simulink library "Lib_HStab"  (R2018b)
settings: Solver=VariableStepAuto  StartTime=0.0  StopTime=10.0  RelTol=1e-3
values from neighbouring files (symbols this model uses):
  AutoTrim_On = 1    [SimulationHStabConfig.m]
  dt = DLLSim.dt    [SimulationTimeStep.m]    (also in SimulationTrim.m = 0.02)
  HStab = 0    [SimulationAircraftConfig.m]
  HStab_Offset = 0    [SimulationHStabConfig.m]
undefined symbols (not defined in the file or in its folder): DiscIntNeverNeededParam, HStabSystem, Trim_REFSI_FD_IN_nmodeStabCmd
libraries: simulink x14, $bdroot x2
settings Model: Creator=JCdFFigueira  LastModifiedBy=JFigueira-Admin
settings DataIOCC: ReturnWorkspaceOutputs=on
settings DebuggingCC: UnconnectedInputMsg=none  UnconnectedOutputMsg=none  UnconnectedLineMsg=none
settings ModelReferenceCC: EnableRefExpFcnMdlSchedulingChecks=off
settings RTWCC: Description=Generic Real-Time Target

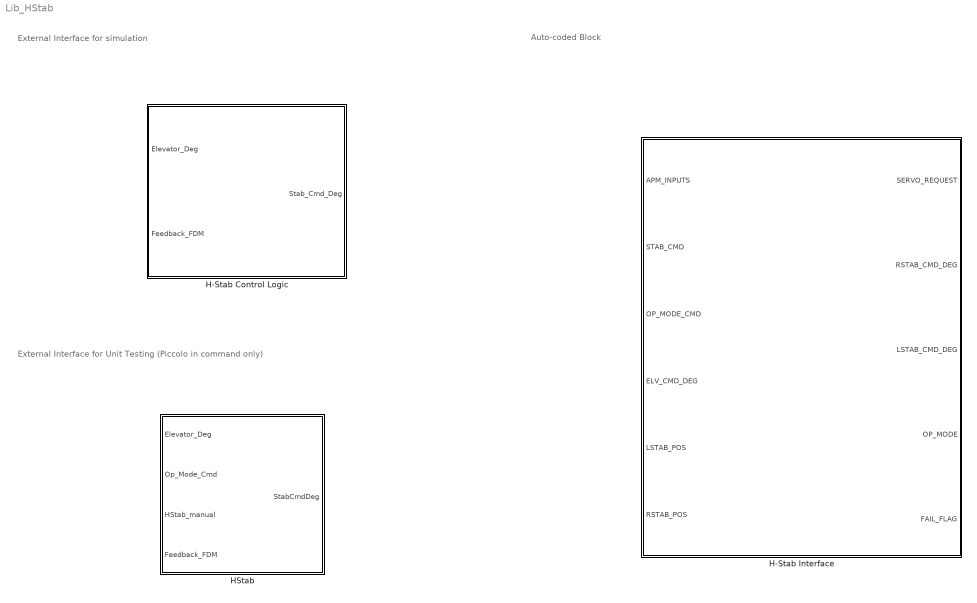
== system Lib_HStab ==
  note: External Interface for Unit Testing (Piccolo in command only)
  note: External Interface for simulation
  note: Auto-coded Block
  H-Stab Control Logic : Subsystem  Variant=on  VariantControl=Variant1
  H-Stab Interface : Subsystem  TreatAsAtomicUnit=on  SystemSampleTime=0.02
  HStab : Subsystem

== system Lib_HStab/H-Stab Control Logic ==
  "Elevator_Deg " : Inport
  Feedback_FDM : Inport  Port=2
  H-Stab Control Logic : Subsystem  VariantControl=FTV == 4 && FDMRelease >= 40
  H-Stab Placeholder : Subsystem  VariantControl=FTV == 3 || FDMRelease < 40
  " Stab_Cmd_Deg" : Outport

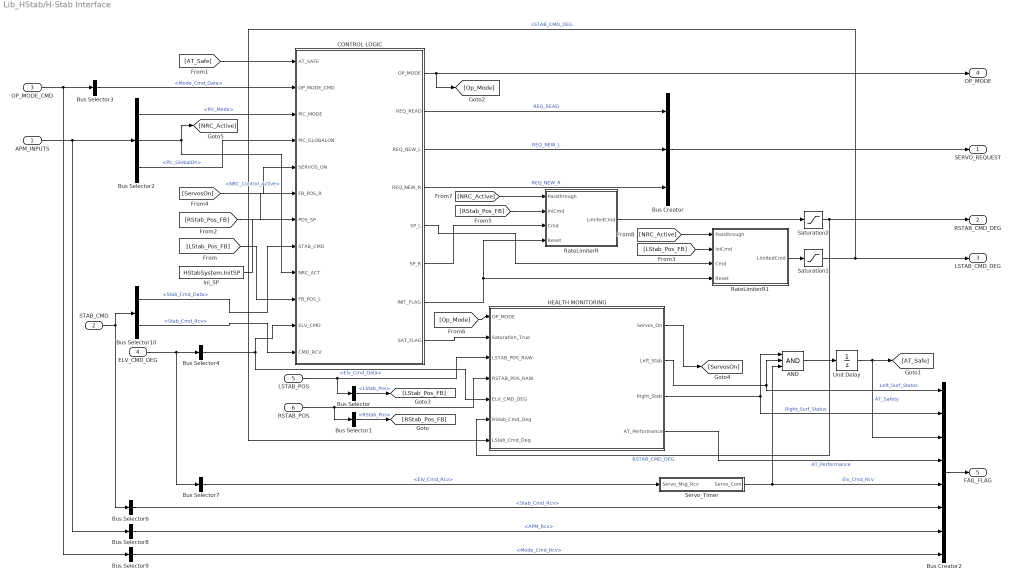
== system Lib_HStab/H-Stab Interface ==
  APM_INPUTS : Inport  OutDataTypeStr=Bus: APM_Bus
  STAB_CMD : Inport  Port=2  OutDataTypeStr=Bus: HStab_Cmd  LockScale=on
  OP_MODE_CMD : Inport  Port=3  OutDataTypeStr=Bus: Mode_Cmd
  ELV_CMD_DEG : Inport  Port=4  OutDataTypeStr=Bus: ELV_Cmd  LockScale=on
  LSTAB_POS : Inport  Port=5  OutDataTypeStr=Bus: LServo_FB  LockScale=on
  RSTAB_POS : Inport  Port=6  OutDataTypeStr=Bus: RServo_FB  LockScale=on
  AND : Logic  Inputs=3  IconShape=distinctive  AllPortsSameDT=off  OutDataTypeStr=boolean
  Bus Creator : BusCreator  Inputs=3
  Bus Creator2 : BusCreator  Inputs=8
  Bus Selector : BusSelector  OutputSignals=LStab_Pos
  Bus Selector1 : BusSelector  OutputSignals=RStab_Pos
  Bus Selector10 : BusSelector  OutputSignals=Stab_Cmd_Data,Stab_Cmd_Rcv
  Bus Selector2 : BusSelector  OutputSignals=Pic_Mode,NRC_Control_Active,Pic_GlobalOn
  Bus Selector3 : BusSelector  OutputSignals=Mode_Cmd_Data
  Bus Selector4 : BusSelector  OutputSignals=Elv_Cmd_Data
  Bus Selector6 : BusSelector  OutputSignals=Stab_Cmd_Rcv
  Bus Selector7 : BusSelector  OutputSignals=Elv_Cmd_Rcv
  Bus Selector8 : BusSelector  OutputSignals=APM_Rcv
  Bus Selector9 : BusSelector  OutputSignals=Mode_Cmd_Rcv
  CONTROL LOGIC : Stateflow chart  TreatAsAtomicUnit=on  SystemSampleTime=0.02
  HEALTH MONITORING : Subsystem
  Ini_SP : Constant  Value=HStabSystem.InitSP  OutDataTypeStr=single
  RateLimiterR : Subsystem
  RateLimiterR1 : Subsystem
  Saturation1 : Saturate  UpperLimit=HStabSystem.LimitUpper  LowerLimit=HStabSystem.LimitLower  OutDataTypeStr=single
  Saturation2 : Saturate  UpperLimit=HStabSystem.LimitUpper  LowerLimit=HStabSystem.LimitLower  OutDataTypeStr=single
  Servo_Timer : Subsystem
  Unit Delay : UnitDelay  InitialCondition=1  SampleTime=0.02
  SERVO_REQUEST : Outport  OutDataTypeStr=Bus: Servo_Request  SampleTime=0.02  VectorParamsAs1DForOutWhenUnconnected=on
  RSTAB_CMD_DEG : Outport  Port=2  OutDataTypeStr=single  VectorParamsAs1DForOutWhenUnconnected=on
  LSTAB_CMD_DEG : Outport  Port=3  OutDataTypeStr=single  VectorParamsAs1DForOutWhenUnconnected=on
  OP_MODE : Outport  Port=4  OutDataTypeStr=uint8  VectorParamsAs1DForOutWhenUnconnected=on
  FAIL_FLAG : Outport  Port=5  OutDataTypeStr=Bus: Fail_Flag_Bus  VectorParamsAs1DForOutWhenUnconnected=on
  wires:
  Saturation1/1 -> LSTAB_CMD_DEG/1, HEALTH MONITORING/7(LStab_Cmd_Deg)  "LSTAB_CMD_DEG"
  Saturation2/1 -> RSTAB_CMD_DEG/1, HEALTH MONITORING/6(RStab_Cmd_Deg)  "RSTAB_CMD_DEG"
  RateLimiterR/1(LimitedCmd) -> Saturation2/1
  [RStab_Pos_FB] -> RateLimiterR/2(IniCmd)
  [LStab_Pos_FB] -> RateLimiterR1/2(IniCmd)
  [RStab_Pos_FB] -> CONTROL LOGIC/6(FB_POS_R)
  [LStab_Pos_FB] -> CONTROL LOGIC/10(FB_POS_L)
  Bus Selector1/1 -> [RStab_Pos_FB]  "<RStab_Pos>"
  Bus Selector/1 -> [LStab_Pos_FB]  "<LStab_Pos>"
  CONTROL LOGIC/7(INIT_FLAG) -> RateLimiterR/4(Reset), RateLimiterR1/4(Reset)
  RateLimiterR1/1(LimitedCmd) -> Saturation1/1
  CONTROL LOGIC/5(SP_L) -> RateLimiterR1/3(Cmd)
  CONTROL LOGIC/6(SP_R) -> RateLimiterR/3(Cmd)
  [ServosOn] -> CONTROL LOGIC/5(SERVOS_ON)
  HEALTH MONITORING/1(Servos_On) -> [ServosOn]
  STAB_CMD/1 -> Bus Selector6/1, Bus Selector10/1
  Ini_SP/1 -> CONTROL LOGIC/7(POS_SP)
  Bus Creator/1 -> SERVO_REQUEST/1
  ELV_CMD_DEG/1 -> Bus Selector7/1, Bus Selector4/1
  CONTROL LOGIC/1(OP_MODE) -> OP_MODE/1, [Op_Mode]
  RSTAB_POS/1 -> HEALTH MONITORING/4(RSTAB_POS_RAW), Bus Selector1/1
  LSTAB_POS/1 -> HEALTH MONITORING/3(LSTAB_POS_RAW), Bus Selector/1
  OP_MODE_CMD/1 -> Bus Selector9/1, Bus Selector3/1
  APM_INPUTS/1 -> Bus Selector8/1, Bus Selector2/1
  HEALTH MONITORING/3(Right_Stab) -> Bus Creator2/2, AND/1  "Right_Surf_Status"
  HEALTH MONITORING/2(Left_Stab) -> Bus Creator2/1, AND/2  "Left_Surf_Status"
  Bus Creator2/1 -> FAIL_FLAG/1
  CONTROL LOGIC/8(SAT_FLAG) -> HEALTH MONITORING/2(Saturation_True)
  HEALTH MONITORING/4(AT_Performance) -> Bus Creator2/4  "AT_Performance"
  Bus Selector2/1 -> CONTROL LOGIC/3(PIC_MODE)  "<Pic_Mode>"
  Bus Selector2/2 -> CONTROL LOGIC/9(NRC_ACT), [NRC_Active]  "<NRC_Control_Active>"
  Bus Selector2/3 -> CONTROL LOGIC/4(PIC_GLOBALON)  "<Pic_GlobalOn>"
  Bus Selector3/1 -> CONTROL LOGIC/2(OP_MODE_CMD)  "<Mode_Cmd_Data>"
  Bus Selector4/1 -> HEALTH MONITORING/5(ELV_CMD_DEG), CONTROL LOGIC/11(ELV_CMD)  "<Elv_Cmd_Data>"
  Bus Selector6/1 -> Bus Creator2/6  "<Stab_Cmd_Rcv>"
  Bus Selector8/1 -> Bus Creator2/7  "<APM_Rcv>"
  Bus Selector9/1 -> Bus Creator2/8  "<Mode_Cmd_Rcv>"
  CONTROL LOGIC/2(REQ_READ) -> Bus Creator/1  "REQ_READ"
  CONTROL LOGIC/3(REQ_NEW_L) -> Bus Creator/2  "REQ_NEW_L"
  CONTROL LOGIC/4(REQ_NEW_R) -> Bus Creator/3  "REQ_NEW_R"
  AND/1 -> Unit Delay/1
  [AT_Safe] -> CONTROL LOGIC/1(AT_SAFE)
  Unit Delay/1 -> Bus Creator2/3, [AT_Safe]  "AT_Safety"
  Bus Selector10/1 -> CONTROL LOGIC/8(STAB_CMD)  "<Stab_Cmd_Data>"
  [Op_Mode] -> HEALTH MONITORING/1(OP_MODE)
  [NRC_Active] -> RateLimiterR/1(Passthrough)
  [NRC_Active] -> RateLimiterR1/1(Passthrough)
  Bus Selector10/2 -> CONTROL LOGIC/12(CMD_RCV)  "<Stab_Cmd_Rcv>"
  Servo_Timer/1(Servo_Com) -> AND/3, Bus Creator2/5  "Elv_Cmd_Rcv"
  Bus Selector7/1 -> Servo_Timer/1(Servo_Msg_Rcv)  "<Elv_Cmd_Rcv>"

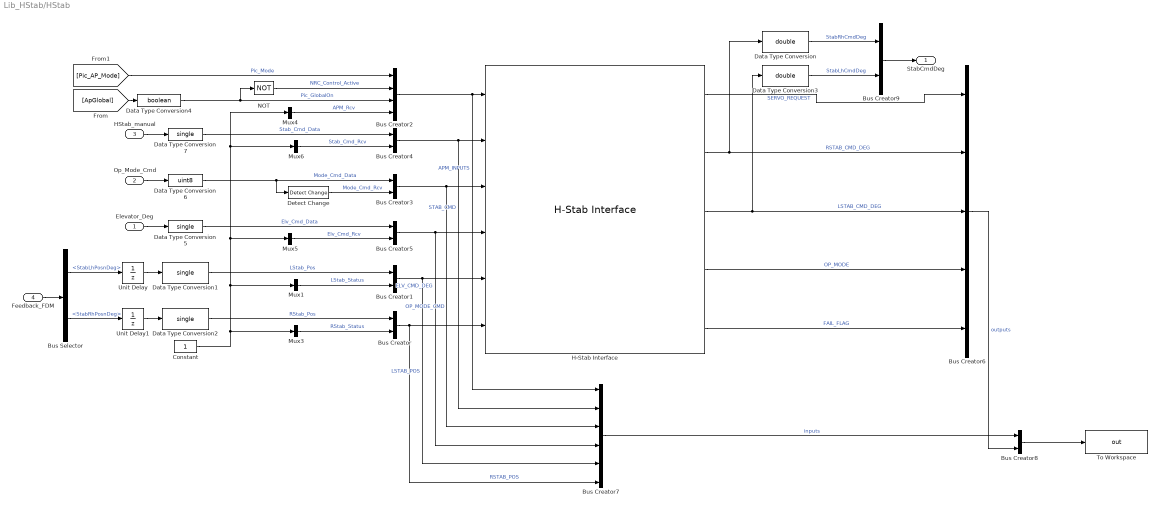
== system Lib_HStab/HStab ==
  Elevator_Deg : Inport  OutDataTypeStr=single  LockScale=on
  Op_Mode_Cmd : Inport  Port=2  OutDataTypeStr=uint8  LockScale=on
  HStab_manual : Inport  Port=3  OutDataTypeStr=single  LockScale=on
  Feedback_FDM : Inport  Port=4
  Bus Creator{,1,3..5,8..9} (7 alike) : BusCreator  Inputs=2
  Bus Creator2 : BusCreator  Inputs=4
  Bus Creator6 : BusCreator  Inputs=5
  Bus Creator7 : BusCreator  Inputs=6
  Bus Selector : BusSelector  OutputSignals=StabLhPosnDeg,StabRhPosnDeg
  Constant : Constant  OutDataTypeStr=boolean
  Data Type Conversion : DataTypeConversion  OutDataTypeStr=double
  Data Type Conversion{1..2,5,7} (4 alike) : DataTypeConversion  OutDataTypeStr=single
  Data Type Conversion3 : DataTypeConversion  OutDataTypeStr=double
  Data Type Conversion4 : DataTypeConversion  OutDataTypeStr=boolean
  Data Type Conversion6 : DataTypeConversion  OutDataTypeStr=uint8
  Detect Change : simulink/Logic and Bit Operations/Detect Change  vinit=2  OutDataTypeStr=boolean
  H-Stab Interface : $bdroot/H-Stab Interface  SystemSampleTime=0.02
  Mux{1,3..6} (5 alike) : Mux  Inputs=1
  NOT : Logic  Operator=NOT  IconShape=distinctive  AllPortsSameDT=off  OutDataTypeStr=boolean
  To Workspace : ToWorkspace  VariableName=out  SaveFormat=Timeseries  SampleTime=dt
  Unit Delay : UnitDelay  InitialCondition=HStab  SampleTime=dt
  Unit Delay1 : UnitDelay  InitialCondition=HStab  SampleTime=dt
  StabCmdDeg : Outport  OutDataTypeStr=double  VectorParamsAs1DForOutWhenUnconnected=on
  wires:
  Data Type Conversion4/1 -> NOT/1, Bus Creator2/3  "Pic_GlobalOn"
  [Pic_AP_Mode] -> Bus Creator2/1  "Pic_Mode"
  Data Type Conversion5/1 -> Bus Creator5/1  "Elv_Cmd_Data"
  Data Type Conversion7/1 -> Bus Creator4/1  "Stab_Cmd_Data"
  Data Type Conversion1/1 -> Bus Creator1/1  "LStab_Pos"
  Mux1/1 -> Bus Creator1/2  "LStab_Status"
  Data Type Conversion2/1 -> Bus Creator/1  "RStab_Pos"
  Mux3/1 -> Bus Creator/2  "RStab_Status"
  Constant/1 -> Mux3/1, Mux1/1, Mux5/1, Mux6/1, Mux4/1
  NOT/1 -> Bus Creator2/2  "NRC_Control_Active"
  Data Type Conversion6/1 -> Detect Change/1, Bus Creator3/1  "Mode_Cmd_Data"
  Mux4/1 -> Bus Creator2/4  "APM_Rcv"
  Mux5/1 -> Bus Creator5/2  "Elv_Cmd_Rcv"
  Mux6/1 -> Bus Creator4/2  "Stab_Cmd_Rcv"
  Detect Change/1 -> Bus Creator3/2  "Mode_Cmd_Rcv"
  Unit Delay/1 -> Data Type Conversion1/1
  H-Stab Interface/2 -> Bus Creator6/2, Data Type Conversion/1  "RSTAB_CMD_DEG"
  H-Stab Interface/1 -> Bus Creator6/1  "SERVO_REQUEST"
  H-Stab Interface/4 -> Bus Creator6/4  "OP_MODE"
  H-Stab Interface/3 -> Bus Creator6/3, Data Type Conversion3/1  "LSTAB_CMD_DEG"
  Bus Creator6/1 -> Bus Creator8/2  "outputs"
  H-Stab Interface/5 -> Bus Creator6/5  "FAIL_FLAG"
  Bus Creator1/1 -> H-Stab Interface/5, Bus Creator7/5  "LSTAB_POS"
  Bus Creator3/1 -> H-Stab Interface/3, Bus Creator7/3  "OP_MODE_CMD"
  Bus Creator5/1 -> H-Stab Interface/4, Bus Creator7/4  "ELV_CMD_DEG"
  Bus Creator4/1 -> H-Stab Interface/2, Bus Creator7/2  "STAB_CMD"
  Bus Creator7/1 -> Bus Creator8/1  "inputs"
  Bus Creator/1 -> H-Stab Interface/6, Bus Creator7/6  "RSTAB_POS"
  Bus Creator2/1 -> H-Stab Interface/1, Bus Creator7/1  "APM_INPUTS"
  Unit Delay1/1 -> Data Type Conversion2/1
  Data Type Conversion/1 -> Bus Creator9/1  "StabRhCmdDeg"
  Data Type Conversion3/1 -> Bus Creator9/2  "StabLhCmdDeg"
  Bus Creator8/1 -> To Workspace/1
  Bus Creator9/1 -> StabCmdDeg/1
  [ApGlobal] -> Data Type Conversion4/1
  Elevator_Deg/1 -> Data Type Conversion5/1
  Op_Mode_Cmd/1 -> Data Type Conversion6/1
  HStab_manual/1 -> Data Type Conversion7/1
  Feedback_FDM/1 -> Bus Selector/1
  Bus Selector/1 -> Unit Delay/1  "<StabLhPosnDeg>"
  Bus Selector/2 -> Unit Delay1/1  "<StabRhPosnDeg>"

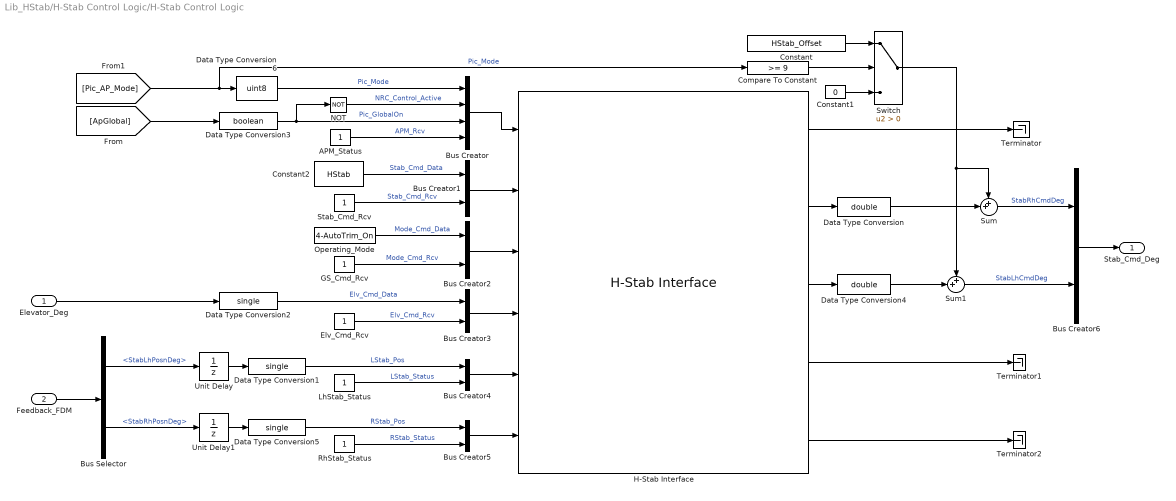
== system Lib_HStab/H-Stab Control Logic/H-Stab Control Logic ==
  Elevator_Deg : Inport
  Feedback_FDM : Inport  Port=2
  APM_Status : Constant  OutDataTypeStr=boolean
  Bus Creator : BusCreator  Inputs=4
  Bus Creator{1..6} (6 alike) : BusCreator  Inputs=2
  Bus Selector : BusSelector  OutputSignals=StabLhPosnDeg,StabRhPosnDeg
  Compare To Constant : simulink/Logic and Bit Operations/Compare To Constant  relop=>=  const=9  OutDataTypeStr=boolean
  Constant : Constant  Value=HStab_Offset  OutDataTypeStr=double
  Constant1 : Constant  Value=0  OutDataTypeStr=double
  Constant2 : Constant  Value=HStab  OutDataTypeStr=single
  Data Type Conversion : DataTypeConversion  OutDataTypeStr=double  LockScale=on
  Data Type Conversion1 : DataTypeConversion  OutDataTypeStr=single
  Data Type Conversion2 : DataTypeConversion  OutDataTypeStr=single
  Data Type Conversion3 : DataTypeConversion  OutDataTypeStr=boolean
  Data Type Conversion4 : DataTypeConversion  OutDataTypeStr=double  LockScale=on
  Data Type Conversion5 : DataTypeConversion  OutDataTypeStr=single
  Data Type Conversion6 : DataTypeConversion  OutDataTypeStr=uint8
  Elv_Cmd_Rcv : Constant  OutDataTypeStr=boolean
  GS_Cmd_Rcv : Constant  OutDataTypeStr=boolean
  H-Stab Interface : $bdroot/H-Stab Interface  SystemSampleTime=0.02
  LhStab_Status : Constant  OutDataTypeStr=boolean
  NOT : Logic  Operator=NOT  IconShape=distinctive  AllPortsSameDT=off  OutDataTypeStr=boolean
  Operating_Mode : Constant  Value=4-AutoTrim_On  OutDataTypeStr=uint8
  RhStab_Status : Constant  OutDataTypeStr=boolean
  Stab_Cmd_Rcv : Constant  OutDataTypeStr=boolean
  Sum : Sum  Inputs=++|
  Sum1 : Sum  Inputs=++|
  Switch : Switch  Criteria=u2 > Threshold
  Terminator : Terminator
  Terminator1 : Terminator
  Terminator2 : Terminator
  Unit Delay : UnitDelay  InitialCondition=HStab  SampleTime=-1
  Unit Delay1 : UnitDelay  InitialCondition=HStab  SampleTime=-1
  Stab_Cmd_Deg : Outport
  wires:
  [Pic_AP_Mode] -> Compare To Constant/1, Data Type Conversion6/1  "Pic_Mode"
  Switch/1 -> Sum1/1, Sum/1
  Compare To Constant/1 -> Switch/2
  Constant/1 -> Switch/1
  Constant1/1 -> Switch/3
  Data Type Conversion6/1 -> Bus Creator/1  "Pic_Mode"
  [ApGlobal] -> Data Type Conversion3/1
  Unit Delay1/1 -> Data Type Conversion5/1
  Bus Selector/2 -> Unit Delay1/1  "<StabRhPosnDeg>"
  Bus Selector/1 -> Unit Delay/1  "<StabLhPosnDeg>"
  H-Stab Interface/4 -> Terminator1/1
  Bus Creator/1 -> H-Stab Interface/1
  Bus Creator4/1 -> H-Stab Interface/5
  APM_Status/1 -> Bus Creator/4  "APM_Rcv"
  RhStab_Status/1 -> Bus Creator5/2  "RStab_Status"
  H-Stab Interface/2 -> Data Type Conversion/1
  Bus Creator1/1 -> H-Stab Interface/2
  Data Type Conversion3/1 -> Bus Creator/3, NOT/1  "Pic_GlobalOn"
  H-Stab Interface/1 -> Terminator/1
  NOT/1 -> Bus Creator/2  "NRC_Control_Active"
  Bus Creator2/1 -> H-Stab Interface/3
  Elv_Cmd_Rcv/1 -> Bus Creator3/2  "Elv_Cmd_Rcv"
  H-Stab Interface/5 -> Terminator2/1
  Bus Creator5/1 -> H-Stab Interface/6
  Data Type Conversion5/1 -> Bus Creator5/1  "RStab_Pos"
  Stab_Cmd_Rcv/1 -> Bus Creator1/2  "Stab_Cmd_Rcv"
  Data Type Conversion1/1 -> Bus Creator4/1  "LStab_Pos"
  Data Type Conversion2/1 -> Bus Creator3/1  "Elv_Cmd_Data"
  Operating_Mode/1 -> Bus Creator2/1  "Mode_Cmd_Data"
  Unit Delay/1 -> Data Type Conversion1/1
  Feedback_FDM/1 -> Bus Selector/1
  GS_Cmd_Rcv/1 -> Bus Creator2/2  "Mode_Cmd_Rcv"
  Elevator_Deg/1 -> Data Type Conversion2/1
  Constant2/1 -> Bus Creator1/1  "Stab_Cmd_Data"
  LhStab_Status/1 -> Bus Creator4/2  "LStab_Status"
  Bus Creator3/1 -> H-Stab Interface/4
  H-Stab Interface/3 -> Data Type Conversion4/1
  Sum/1 -> Bus Creator6/1  "StabRhCmdDeg"
  Sum1/1 -> Bus Creator6/2  "StabLhCmdDeg"
  Bus Creator6/1 -> Stab_Cmd_Deg/1
  Data Type Conversion4/1 -> Sum1/2
  Data Type Conversion/1 -> Sum/2

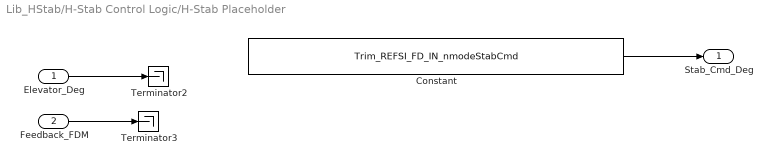
== system Lib_HStab/H-Stab Control Logic/H-Stab Placeholder ==
  Elevator_Deg : Inport
  Feedback_FDM : Inport  Port=2
  Constant : Constant  Value=Trim_REFSI_FD_IN_nmodeStabCmd
  Terminator2 : Terminator
  Terminator3 : Terminator
  Stab_Cmd_Deg : Outport
  wires:
  Constant/1 -> Stab_Cmd_Deg/1
  Elevator_Deg/1 -> Terminator2/1
  Feedback_FDM/1 -> Terminator3/1

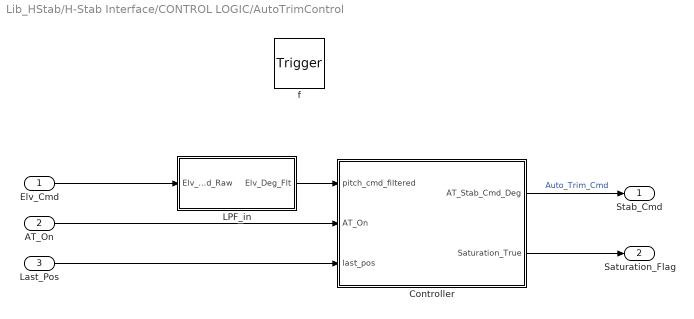
== system Lib_HStab/H-Stab Interface/CONTROL LOGIC/AutoTrimControl ==
  Elv_Cmd : Inport  OutDataTypeStr=single  PortDimensions=1
  AT_On : Inport  Port=2  OutDataTypeStr=boolean  PortDimensions=1
  Last_Pos : Inport  Port=3  OutDataTypeStr=single  PortDimensions=1
  f : TriggerPort  TriggerType=function-call  VariantControl=(inherit)
      settings: CopyFcn=Stateflow.SLINSF.SimulinkMan.removeBlockPreDeleteFcn  PreDeleteFcn=Stateflow.SLINSF.SimulinkMan.unsafePredeleteFcn
  "Controller " : Subsystem
  LPF_in : Subsystem
  Stab_Cmd : Outport  OutDataTypeStr=single  PortDimensions=1  VectorParamsAs1DForOutWhenUnconnected=on
  Saturation_Flag : Outport  Port=2  OutDataTypeStr=boolean  PortDimensions=1  VectorParamsAs1DForOutWhenUnconnected=on
  wires:
  "Controller "/2(Saturation_True) -> Saturation_Flag/1
  "Controller "/1(AT_Stab_Cmd_Deg) -> Stab_Cmd/1  "Auto_Trim_Cmd"
  Last_Pos/1 -> "Controller "/3(last_pos)
  LPF_in/1(Elv_Deg_Flt) -> "Controller "/1(pitch_cmd_filtered)
  AT_On/1 -> "Controller "/2(AT_On)
  Elv_Cmd/1 -> LPF_in/1(Elv_Cmd_Raw)

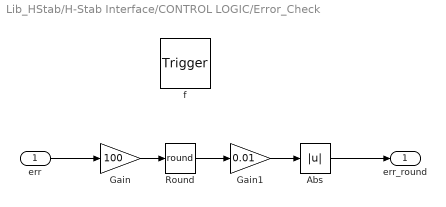
== system Lib_HStab/H-Stab Interface/CONTROL LOGIC/Error_Check ==
  err : Inport  OutDataTypeStr=single  PortDimensions=1
  f : TriggerPort  TriggerType=function-call  VariantControl=(inherit)
      settings: CopyFcn=Stateflow.SLINSF.SimulinkMan.removeBlockPreDeleteFcn  PreDeleteFcn=Stateflow.SLINSF.SimulinkMan.unsafePredeleteFcn
  Abs : Abs  OutDataTypeStr=single
  Gain : Gain  Gain=100
  Gain1 : Gain  Gain=0.01
  Round : Rounding  Operator=round
  err_round : Outport  OutDataTypeStr=single  PortDimensions=1  VectorParamsAs1DForOutWhenUnconnected=on
  wires:
  Round/1 -> Gain1/1
  Gain/1 -> Round/1
  Gain1/1 -> Abs/1
  err/1 -> Gain/1
  Abs/1 -> err_round/1

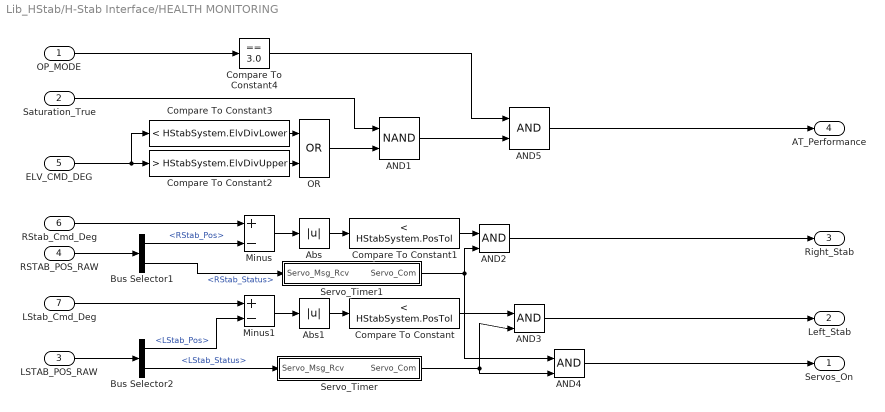
== system Lib_HStab/H-Stab Interface/HEALTH MONITORING ==
  OP_MODE : Inport  PortDimensions=1
  Saturation_True : Inport  Port=2  OutDataTypeStr=boolean  PortDimensions=1
  LSTAB_POS_RAW : Inport  Port=3  OutDataTypeStr=Bus: LServo_FB
  RSTAB_POS_RAW : Inport  Port=4  OutDataTypeStr=Bus: RServo_FB
  ELV_CMD_DEG : Inport  Port=5  OutDataTypeStr=single  PortDimensions=1
  RStab_Cmd_Deg : Inport  Port=6  OutDataTypeStr=single  PortDimensions=1
  LStab_Cmd_Deg : Inport  Port=7  OutDataTypeStr=single  PortDimensions=1
  AND1 : Logic  Operator=NAND  IconShape=distinctive  AllPortsSameDT=off  OutDataTypeStr=boolean
  AND{2..5} (4 alike) : Logic  IconShape=distinctive  AllPortsSameDT=off  OutDataTypeStr=boolean
  Abs : Abs  OutDataTypeStr=single
  Abs1 : Abs  OutDataTypeStr=single
  Bus Selector1 : BusSelector  OutputSignals=RStab_Pos,RStab_Status
  Bus Selector2 : BusSelector  OutputSignals=LStab_Pos,LStab_Status
  Compare To Constant : simulink/Logic and Bit Operations/Compare To Constant  relop=<  const=HStabSystem.PosTol  OutDataTypeStr=boolean
  Compare To Constant1 : simulink/Logic and Bit Operations/Compare To Constant  relop=<  const=HStabSystem.PosTol  OutDataTypeStr=boolean
  Compare To Constant2 : simulink/Logic and Bit Operations/Compare To Constant  relop=>  const=HStabSystem.ElvDivUpper  OutDataTypeStr=boolean
  Compare To Constant3 : simulink/Logic and Bit Operations/Compare To Constant  relop=<  const=HStabSystem.ElvDivLower  OutDataTypeStr=boolean
  Compare To Constant4 : simulink/Logic and Bit Operations/Compare To Constant  relop===  const=3.0  OutDataTypeStr=boolean
  Minus : Sum  Inputs=+-
  Minus1 : Sum  Inputs=+-
  OR : Logic  Operator=OR  IconShape=distinctive  AllPortsSameDT=off  OutDataTypeStr=boolean
  Servo_Timer : Subsystem
  Servo_Timer1 : Subsystem
  Servos_On : Outport  OutDataTypeStr=boolean  PortDimensions=1  VectorParamsAs1DForOutWhenUnconnected=on
  Left_Stab : Outport  Port=2  OutDataTypeStr=boolean  PortDimensions=1  VectorParamsAs1DForOutWhenUnconnected=on
  Right_Stab : Outport  Port=3  OutDataTypeStr=boolean  PortDimensions=1  VectorParamsAs1DForOutWhenUnconnected=on
  AT_Performance : Outport  Port=4  OutDataTypeStr=boolean  PortDimensions=1  VectorParamsAs1DForOutWhenUnconnected=on
  wires:
  Bus Selector1/2 -> Servo_Timer1/1(Servo_Msg_Rcv)  "<RStab_Status>"
  Bus Selector2/2 -> Servo_Timer/1(Servo_Msg_Rcv)  "<LStab_Status>"
  Servo_Timer/1(Servo_Com) -> AND4/2, AND3/2
  AND4/1 -> Servos_On/1
  LStab_Cmd_Deg/1 -> Minus1/1
  RStab_Cmd_Deg/1 -> Minus/1
  Servo_Timer1/1(Servo_Com) -> AND4/1, AND2/2
  LSTAB_POS_RAW/1 -> Bus Selector2/1
  RSTAB_POS_RAW/1 -> Bus Selector1/1
  Compare To Constant/1 -> AND3/1
  Compare To Constant1/1 -> AND2/1
  Abs1/1 -> Compare To Constant/1
  Abs/1 -> Compare To Constant1/1
  Minus/1 -> Abs/1
  Minus1/1 -> Abs1/1
  Bus Selector2/1 -> Minus1/2  "<LStab_Pos>"
  Bus Selector1/1 -> Minus/2  "<RStab_Pos>"
  OR/1 -> AND1/2
  Compare To Constant3/1 -> OR/1
  Compare To Constant2/1 -> OR/2
  ELV_CMD_DEG/1 -> Compare To Constant2/1, Compare To Constant3/1
  Saturation_True/1 -> AND1/1
  AND1/1 -> AND5/2
  AND3/1 -> Left_Stab/1
  AND2/1 -> Right_Stab/1
  OP_MODE/1 -> Compare To Constant4/1
  Compare To Constant4/1 -> AND5/1
  AND5/1 -> AT_Performance/1

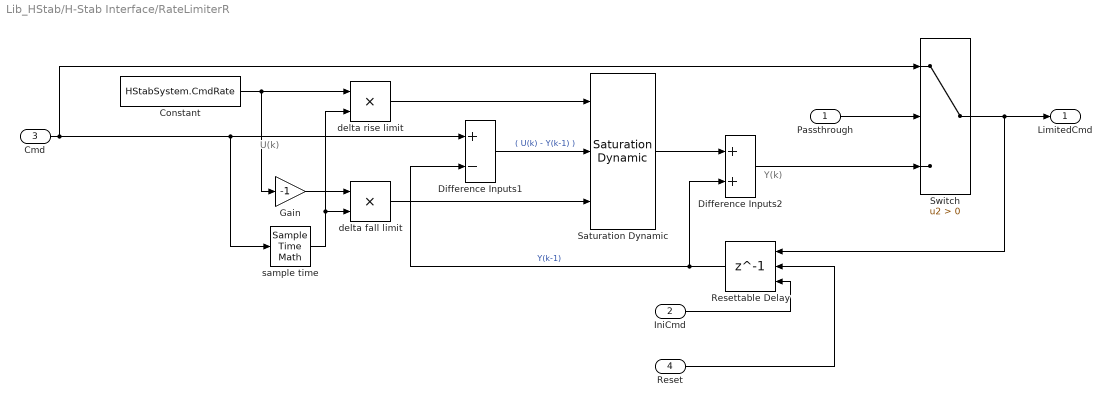
== system Lib_HStab/H-Stab Interface/RateLimiterR ==
  note: Y(k)
  note: U(k)
  Passthrough : Inport  OutDataTypeStr=boolean  PortDimensions=1
  IniCmd : Inport  Port=2  OutDataTypeStr=single  PortDimensions=1
  Cmd : Inport  Port=3  OutDataTypeStr=single  PortDimensions=1
  Reset : Inport  Port=4  OutDataTypeStr=boolean  PortDimensions=1
  Constant : Constant  Value=HStabSystem.CmdRate
  Difference Inputs1 : Sum  Description=Add in CPU  DisableCoverage=on  Inputs=+-  OutDataTypeStr=Inherit: Inherit via back propagation
  Difference Inputs2 : Sum  Description=Add in CPU  OutDataTypeStr=Inherit: Inherit via back propagation
  Gain : Gain  Gain=-1
  Resettable Delay : Delay  DelayLength=1  InitialConditionSource=Input port  ExternalReset=Rising  SampleTime=0.02
      settings: InputPortMap=u0,r5,p4
  Saturation Dynamic : simulink/Discontinuities/Saturation Dynamic  OutMin=[]  OutMax=[]  OutDataTypeStr=Inherit: Same as second input  OutDataType=fixdt(1, 16)  OutScaling=2^-10  DoSatur=off
  Switch : Switch  Criteria=u2 > Threshold
  delta fall limit : Product  DisableCoverage=on  Inputs=**  OutDataTypeStr=Inherit: Inherit via back propagation  SaturateOnIntegerOverflow=on
  delta rise limit : Product  DisableCoverage=on  Inputs=**  OutDataTypeStr=Inherit: Inherit via back propagation  SaturateOnIntegerOverflow=on
  sample time : SampleTimeMath  DisableCoverage=on  TsampMathOp=Ts Only  weightValue=1
  LimitedCmd : Outport  OutDataTypeStr=single  PortDimensions=1  VectorParamsAs1DForOutWhenUnconnected=on
  wires:
  Reset/1 -> Resettable Delay/2
  Cmd/1 -> sample time/1, Difference Inputs1/1, Switch/1
  delta rise limit/1 -> Saturation Dynamic/1
  IniCmd/1 -> Resettable Delay/3
  Constant/1 -> delta rise limit/1, Gain/1
  sample time/1 -> delta rise limit/2, delta fall limit/2
  Difference Inputs1/1 -> Saturation Dynamic/2  "( U(k) - Y(k-1) )"
  Saturation Dynamic/1 -> Difference Inputs2/1
  Switch/1 -> Resettable Delay/1, LimitedCmd/1
  Gain/1 -> delta fall limit/1
  Resettable Delay/1 -> Difference Inputs1/2, Difference Inputs2/2  "Y(k-1)"
  delta fall limit/1 -> Saturation Dynamic/3
  Passthrough/1 -> Switch/2
  Difference Inputs2/1 -> Switch/3

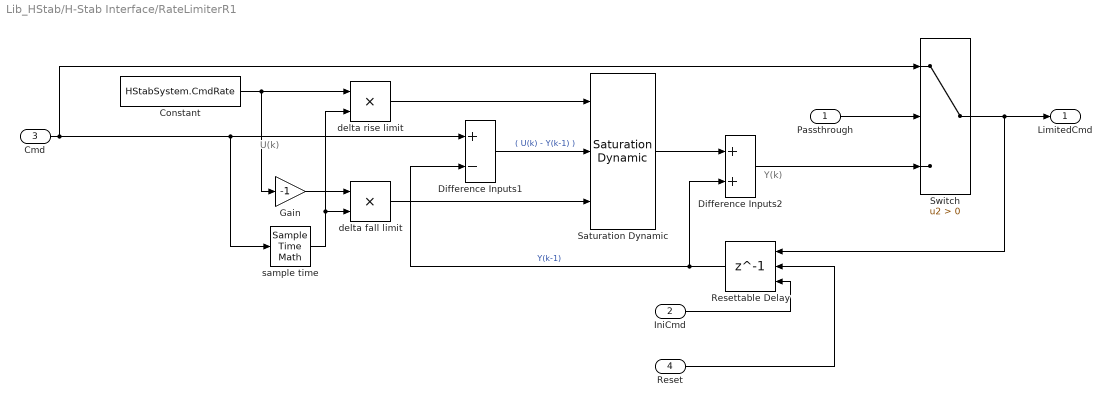
== system Lib_HStab/H-Stab Interface/RateLimiterR1 ==
  note: Y(k)
  note: U(k)
  Passthrough : Inport  OutDataTypeStr=boolean  PortDimensions=1
  IniCmd : Inport  Port=2  OutDataTypeStr=single  PortDimensions=1
  Cmd : Inport  Port=3  OutDataTypeStr=single  PortDimensions=1
  Reset : Inport  Port=4  OutDataTypeStr=boolean  PortDimensions=1
  Constant : Constant  Value=HStabSystem.CmdRate
  Difference Inputs1 : Sum  Description=Add in CPU  DisableCoverage=on  Inputs=+-  OutDataTypeStr=Inherit: Inherit via back propagation
  Difference Inputs2 : Sum  Description=Add in CPU  OutDataTypeStr=Inherit: Inherit via back propagation
  Gain : Gain  Gain=-1
  Resettable Delay : Delay  DelayLength=1  InitialConditionSource=Input port  ExternalReset=Rising  SampleTime=0.02
      settings: InputPortMap=u0,r5,p4
  Saturation Dynamic : simulink/Discontinuities/Saturation Dynamic  OutMin=[]  OutMax=[]  OutDataTypeStr=Inherit: Same as second input  OutDataType=fixdt(1, 16)  OutScaling=2^-10  DoSatur=off
  Switch : Switch  Criteria=u2 > Threshold
  delta fall limit : Product  DisableCoverage=on  Inputs=**  OutDataTypeStr=Inherit: Inherit via back propagation  SaturateOnIntegerOverflow=on
  delta rise limit : Product  DisableCoverage=on  Inputs=**  OutDataTypeStr=Inherit: Inherit via back propagation  SaturateOnIntegerOverflow=on
  sample time : SampleTimeMath  DisableCoverage=on  TsampMathOp=Ts Only  weightValue=1
  LimitedCmd : Outport  OutDataTypeStr=single  PortDimensions=1  VectorParamsAs1DForOutWhenUnconnected=on
  wires:
  Reset/1 -> Resettable Delay/2
  Cmd/1 -> sample time/1, Difference Inputs1/1, Switch/1
  delta rise limit/1 -> Saturation Dynamic/1
  IniCmd/1 -> Resettable Delay/3
  Constant/1 -> delta rise limit/1, Gain/1
  sample time/1 -> delta rise limit/2, delta fall limit/2
  Difference Inputs1/1 -> Saturation Dynamic/2  "( U(k) - Y(k-1) )"
  Saturation Dynamic/1 -> Difference Inputs2/1
  Switch/1 -> Resettable Delay/1, LimitedCmd/1
  Gain/1 -> delta fall limit/1
  Resettable Delay/1 -> Difference Inputs1/2, Difference Inputs2/2  "Y(k-1)"
  delta fall limit/1 -> Saturation Dynamic/3
  Passthrough/1 -> Switch/2
  Difference Inputs2/1 -> Switch/3

== system Lib_HStab/H-Stab Interface/Servo_Timer ==
  Servo_Msg_Rcv : Inport
  Compare To Constant6 : simulink/Logic and Bit Operations/Compare To Constant  relop=<=  const=HStabSystem.ServoTimeout  OutDataTypeStr=boolean
  Discrete-Time Integrator : DiscreteIntegrator  ExternalReset=level  SampleTime=0.02  OutDataTypeStr=single  LimitOutput=on  UpperSaturationLimit=HStabSystem.ServoTimeout+0.1  LowerSaturationLimit=0  ICPrevOutput=DiscIntNeverNeededParam  ICPrevScaledInput=DiscIntNeverNeededParam
  NOT : Logic  Operator=NOT  IconShape=distinctive  AllPortsSameDT=off  OutDataTypeStr=boolean
  Servo_Com : Outport  VectorParamsAs1DForOutWhenUnconnected=on
  wires:
  Servo_Msg_Rcv/1 -> NOT/1, Discrete-Time Integrator/2
  Compare To Constant6/1 -> Servo_Com/1
  NOT/1 -> Discrete-Time Integrator/1
  Discrete-Time Integrator/1 -> Compare To Constant6/1

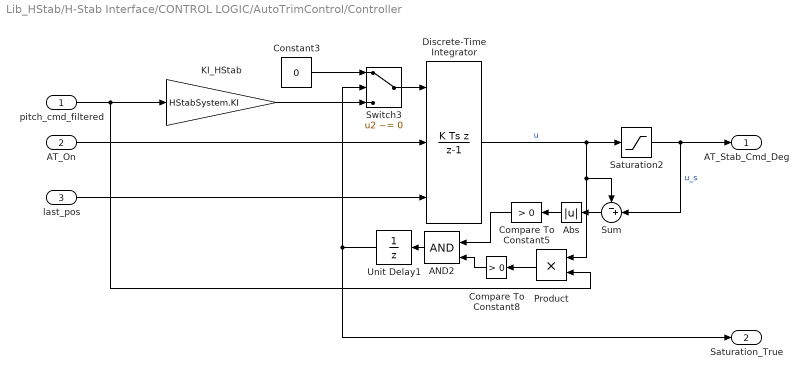
== system Lib_HStab/H-Stab Interface/CONTROL LOGIC/AutoTrimControl/Controller  ==
  pitch_cmd_filtered : Inport  OutDataTypeStr=single
  AT_On : Inport  Port=2
  last_pos : Inport  Port=3  OutDataTypeStr=single
  AND2 : Logic  IconShape=distinctive  AllPortsSameDT=off  OutDataTypeStr=boolean
  Abs : Abs  OutDataTypeStr=single
  Compare To Constant5 : simulink/Logic and Bit Operations/Compare To Constant  relop=>  const=0  OutDataTypeStr=boolean
  Compare To Constant8 : simulink/Logic and Bit Operations/Compare To Constant  relop=>  const=0  OutDataTypeStr=boolean
  Constant3 : Constant  Value=0  OutDataTypeStr=single
  Discrete-Time Integrator : DiscreteIntegrator  IntegratorMethod=Integration: Backward Euler  ExternalReset=rising  InitialConditionSource=external  SampleTime=-1  OutDataTypeStr=single  ICPrevOutput=DiscIntNeverNeededParam  ICPrevScaledInput=DiscIntNeverNeededParam
  KI_HStab : Gain  Gain=HStabSystem.KI  OutDataTypeStr=single
  Product : Product  OutDataTypeStr=single
  Saturation2 : Saturate  UpperLimit=HStabSystem.LimitUpper  LowerLimit=HStabSystem.LimitLower  OutDataTypeStr=single
  Sum : Sum  Inputs=-+|  AccumDataTypeStr=single  OutDataTypeStr=single
  Switch3 : Switch  Criteria=u2 ~= 0  OutDataTypeStr=single
  Unit Delay1 : UnitDelay  SampleTime=-1
  AT_Stab_Cmd_Deg : Outport  OutDataTypeStr=single  PortDimensions=1  VectorParamsAs1DForOutWhenUnconnected=on
  Saturation_True : Outport  Port=2  OutDataTypeStr=boolean  PortDimensions=1  VectorParamsAs1DForOutWhenUnconnected=on
  wires:
  Abs/1 -> Compare To Constant5/1
  last_pos/1 -> Discrete-Time Integrator/3
  Saturation2/1 -> Sum/2, AT_Stab_Cmd_Deg/1  "u_s"
  Unit Delay1/1 -> Saturation_True/1, Switch3/2
  Discrete-Time Integrator/1 -> Product/1, Sum/1, Saturation2/1  "u"
  AND2/1 -> Unit Delay1/1
  Constant3/1 -> Switch3/1
  Product/1 -> Compare To Constant8/1
  Compare To Constant5/1 -> AND2/1
  pitch_cmd_filtered/1 -> KI_HStab/1, Product/2
  KI_HStab/1 -> Switch3/3
  Compare To Constant8/1 -> AND2/2
  Sum/1 -> Abs/1
  Switch3/1 -> Discrete-Time Integrator/1
  AT_On/1 -> Discrete-Time Integrator/2

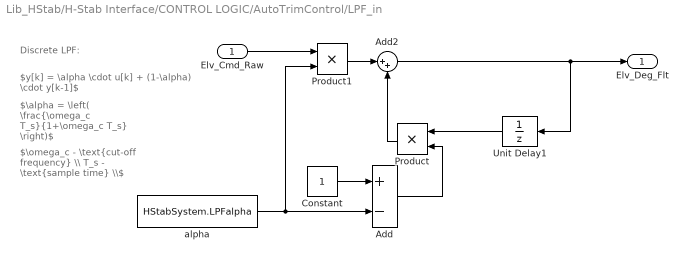
== system Lib_HStab/H-Stab Interface/CONTROL LOGIC/AutoTrimControl/LPF_in ==
  note: $y[k] = \alpha \cdot u[k] + (1-\alpha) \cdot y[k-1]$
  note: Discrete LPF:
  note: $\alpha = \left( \frac{\omega_c T_s}{1+\omega_c T_s} \right)$
  note: $\omega_c - \text{cut-off frequency} \\ T_s - \text{sample time} \\$
  Elv_Cmd_Raw : Inport  OutDataTypeStr=single  PortDimensions=1
  Add : Sum  Inputs=+-  AccumDataTypeStr=single  OutDataTypeStr=single
  Add2 : Sum  Inputs=|++  AccumDataTypeStr=single  OutDataTypeStr=single
  Constant : Constant  OutDataTypeStr=single
  Product : Product  OutDataTypeStr=single
  Product1 : Product  OutDataTypeStr=single
  Unit Delay1 : UnitDelay  SampleTime=-1
  alpha : Constant  Value=HStabSystem.LPFalpha  OutDataTypeStr=single
  Elv_Deg_Flt : Outport  OutDataTypeStr=single  PortDimensions=1  VectorParamsAs1DForOutWhenUnconnected=on
  wires:
  Product/1 -> Add2/2
  Product1/1 -> Add2/1
  Add2/1 -> Unit Delay1/1, Elv_Deg_Flt/1
  alpha/1 -> Add/2, Product1/2
  Add/1 -> Product/2
  Constant/1 -> Add/1
  Unit Delay1/1 -> Product/1
  Elv_Cmd_Raw/1 -> Product1/1

== system Lib_HStab/H-Stab Interface/HEALTH MONITORING/Servo_Timer ==
  Servo_Msg_Rcv : Inport
  Compare To Constant6 : simulink/Logic and Bit Operations/Compare To Constant  relop=<=  const=HStabSystem.ServoTimeout  OutDataTypeStr=boolean
  Discrete-Time Integrator : DiscreteIntegrator  ExternalReset=level  SampleTime=0.02  OutDataTypeStr=single  LimitOutput=on  UpperSaturationLimit=HStabSystem.ServoTimeout+0.1  LowerSaturationLimit=0  ICPrevOutput=DiscIntNeverNeededParam  ICPrevScaledInput=DiscIntNeverNeededParam
  NOT : Logic  Operator=NOT  IconShape=distinctive  AllPortsSameDT=off  OutDataTypeStr=boolean
  Servo_Com : Outport  VectorParamsAs1DForOutWhenUnconnected=on
  wires:
  Servo_Msg_Rcv/1 -> NOT/1, Discrete-Time Integrator/2
  Compare To Constant6/1 -> Servo_Com/1
  NOT/1 -> Discrete-Time Integrator/1
  Discrete-Time Integrator/1 -> Compare To Constant6/1

== system Lib_HStab/H-Stab Interface/HEALTH MONITORING/Servo_Timer1 ==
  Servo_Msg_Rcv : Inport
  Compare To Constant6 : simulink/Logic and Bit Operations/Compare To Constant  relop=<=  const=HStabSystem.ServoTimeout  OutDataTypeStr=boolean
  Discrete-Time Integrator : DiscreteIntegrator  ExternalReset=level  SampleTime=0.02  OutDataTypeStr=single  LimitOutput=on  UpperSaturationLimit=HStabSystem.ServoTimeout+0.1  LowerSaturationLimit=0  ICPrevOutput=DiscIntNeverNeededParam  ICPrevScaledInput=DiscIntNeverNeededParam
  NOT : Logic  Operator=NOT  IconShape=distinctive  AllPortsSameDT=off  OutDataTypeStr=boolean
  Servo_Com : Outport  VectorParamsAs1DForOutWhenUnconnected=on
  wires:
  Servo_Msg_Rcv/1 -> NOT/1, Discrete-Time Integrator/2
  Compare To Constant6/1 -> Servo_Com/1
  NOT/1 -> Discrete-Time Integrator/1
  Discrete-Time Integrator/1 -> Compare To Constant6/1

== stateflow chart Lib_HStab/H-Stab Interface/CONTROL LOGIC ==
  settings: updateMethod=DISCRETE  sampleTime=0.02
  state Servo_Msg_Rcv
    state Flying_Modes
      du: REQ_READ = true; REQ_NEW_R = true; REQ_NEW_L = true;
      (history)
      state AUTOTRIM
        Mode
        [SP_R,SAT_FLAG] = AutoTrimControl(ELV_CMD,IntegralOn,FB_POS_R);
        SP_L = SP_R;
      state DIRECT
        Mode
        SP_R = STAB_CMD;
        SP_L = STAB_CMD;
      state LOCKED
        Mode
        SP_L = Last_SP_L;
        SP_R = Last_SP_R;
      DIRECT -> LOCKED [order 2] : [OP_MODE == 2]{Last_SP_R = FB_POS_R; Last_SP_L = FB_POS_L; }
      (default) -> LOCKED : {Last_SP_R = FB_POS_R; Last_SP_L = FB_POS_L;}
      DIRECT -> AUTOTRIM [order 3] : [OP_MODE == 3]{IntegralOn = false;}
      LOCKED -> AUTOTRIM [order 3] : [OP_MODE == 3]{IntegralOn = false;}
      DIRECT -> DIRECT [order 1] : [OP_MODE == 4]
      AUTOTRIM -> DIRECT [order 2] : [OP_MODE == 4]
      AUTOTRIM -> LOCKED [order 1] : [OP_MODE == 2]{Last_SP_R = SP_R; Last_SP_L = SP_L;}
      LOCKED -> LOCKED [order 1] : [OP_MODE == 2]
      LOCKED -> DIRECT [order 2] : [OP_MODE == 4]
      AUTOTRIM -> AUTOTRIM [order 3] : [OP_MODE == 3]{IntegralOn = true;}
    state INITIALIZATION
      en: REQ_READ = true; REQ_NEW_R = false; REQ_NEW_L = false; INIT_FLAG = true;
      du: OP_MODE = 1;
      ex: INIT_FLAG = false;
      state Right [parallel]
        settings: executionOrder=1
        state POS_Track
          en: pos_err_R = Error_Check(FB_POS_R-INI_SP_R);
        state POS_Correction
          en: REQ_NEW_R = true;
          ex: SP_R = INI_SP_R;
        (default) -> Servo_Msg_Rcv.INITIALIZATION.Right.POS_Track : {SP_R = FB_POS_R;}
        Servo_Msg_Rcv.INITIALIZATION.Right.POS_Track -> Servo_Msg_Rcv.INITIALIZATION.Right.POS_Correction : [pos_err_R > 0]
        Servo_Msg_Rcv.INITIALIZATION.Right.POS_Correction -> Servo_Msg_Rcv.INITIALIZATION.Right.POS_Track : [pos_err_R > 0]
      state Left [parallel]
        settings: executionOrder=2
        state POS_Track
          en: pos_err_L = Error_Check(FB_POS_L-INI_SP_L);
        state POS_Correction
          en: REQ_NEW_L = true;
          ex: SP_L = INI_SP_L;
        (default) -> Servo_Msg_Rcv.INITIALIZATION.Left.POS_Track : {SP_L = FB_POS_L;}
        Servo_Msg_Rcv.INITIALIZATION.Left.POS_Track -> Servo_Msg_Rcv.INITIALIZATION.Left.POS_Correction : [pos_err_L > 0]
        Servo_Msg_Rcv.INITIALIZATION.Left.POS_Correction -> Servo_Msg_Rcv.INITIALIZATION.Left.POS_Track : [pos_err_L > 0]
    (default) -> (junction 733)
    (junction 733) -> (junction 734) [order 1] : [PIC_MODE ~= 0]
    (junction 733) -> (junction 735) [order 2]
    (junction 734) -> (junction 736) : {INI_SP_L = FB_POS_L; INI_SP_R = FB_POS_R;}
    (junction 736) -> (junction 735)
    (junction 735) -> INITIALIZATION
    INITIALIZATION -> Flying_Modes : [pos_err_R < 0.2 && pos_err_L < 0.2 && after(0.04,'sec') ]
  state IDLE
    en: OP_MODE = 0;
    du: REQ_READ = true; REQ_NEW_R = false; REQ_NEW_L = false;
  state err_round = Error_Check(err) [function]
  state [Stab_Cmd,Saturation_Flag] = AutoTrimControl(Elv_Cmd,AT_On,Last_Pos) [function]
  (default) -> IDLE : {INI_SP_R = POS_SP; INI_SP_L = POS_SP}
  IDLE -> Servo_Msg_Rcv : [SERVOS_ON == 1 && after(0.04,'sec')]
  Servo_Msg_Rcv -> IDLE : [SERVOS_ON == 0]/{INI_SP_R = FB_POS_R; INI_SP_L = FB_POS_L}
  data: err function_input single size=1; err_round function_output single size=1; Elv_Cmd function_input single size=1; AT_On function_input boolean size=1; Last_Pos function_input single size=1; Stab_Cmd function_output single size=1; Saturation_Flag function_output boolean size=1; AT_SAFE input boolean; OP_MODE_CMD input uint8 size=1; PIC_MODE input uint8; PIC_GLOBALON input boolean; SERVOS_ON input boolean; OP_MODE output uint8 size=1; FB_POS_R input single; POS_SP input single; STAB_CMD input; NRC_ACT input boolean; REQ_READ output boolean; REQ_NEW_L output boolean; REQ_NEW_R output boolean; FB_POS_L input single; pos_err_L local single; pos_err_R local single; SP_L output single; SP_R output single; INIT_FLAG output boolean; ELV_CMD input; SAT_FLAG output; INI_SP_R local; INI_SP_L local; Last_SP_L local; Last_SP_R local; CMD_RCV input; IntegralOn local
  function Mode:
    | function Mode
    | 
    | aVarTruthTableCondition_1 = false;
    | aVarTruthTableCondition_2 = false;
    | aVarTruthTableCondition_3 = false;
    | aVarTruthTableCondition_4 = false;
    | aVarTruthTableCondition_5 = false;
    | aVarTruthTableCondition_6 = false;
    | aVarTruthTableCondition_7 = false;
    | aVarTruthTableCondition_8 = false;
    | aVarTruthTableCondition_9 = false;
    | 
    | 
    | % NRC in control
    | 
    | aVarTruthTableCondition_1 = logical(NRC_ACT == 1);
    | 
    | % On ground
    | 
    | aVarTruthTableCondition_2 = logical(PIC_MODE == 0);
    | 
    | % Take-off
    | 
    | aVarTruthTableCondition_3 = logical(PIC_MODE <= 3);
    | 
    | % Landing
    | 
    | aVarTruthTableCondition_4 = logical(PIC_MODE >= 9);
    | 
    | % GS command to lock
    | 
    | aVarTruthTableCondition_5 = logical(OP_MODE_CMD == 2);
    | 
    | % GS command to change position
    | 
    | aVarTruthTableCondition_6 = logical(OP_MODE_CMD == 4);
    | 
    | % Rcv Stab Command
    | 
    | aVarTruthTableCondition_7 = logical(CMD_RCV == 1);
    | 
    | % GS command to enable auto-trim
    | 
    | aVarTruthTableCondition_8 = logical(OP_MODE_CMD == 3);
    | 
    | % Safe to use Auto-Trim
    | 
    | aVarTruthTableCondition_9 = logical(AT_SAFE == 1);
    | 
    | if (aVarTruthTableCondition_1 && ~aVarTruthTableCondition_7)
    |     aFcnTruthTableAction_1();
    | elseif (aVarTruthTableCondition_1 && aVarTruthTableCondition_7)
    |     aFcnTruthTableAction_3();
    | elseif (~aVarTruthTableCondition_1 && aVarTruthTableCondition_2 && aVarTruthTableCondition_3 && ~aVarTruthTableCondition_4 && aVarTruthTableCondition_5 && ~aVarTruthTableCondition_6 && ~aVarTruthTableCondition_8)
    |     aFcnTruthTableAction_1();
    | elseif (~aVarTruthTableCondition_1 && aVarTruthTableCondition_2 && aVarTruthTableCondition_3 && ~aVarTruthTableCondition_4 && ~aVarTruthTableCondition_5 && aVarTruthTableCondition_6 && ~aVarTruthTableCondition_8)
    |     aFcnTruthTableAction_3();
    | elseif (~aVarTruthTableCondition_1 && aVarTruthTableCondition_2 && aVarTruthTableCondition_3 && ~aVarTruthTableCondition_4 && ~aVarTruthTableCondition_5 && ~aVarTruthTableCondition_6 && aVarTruthTableCondition_8)
    |     aFcnTruthTableAction_1();
    | elseif (~aVarTruthTableCondition_1 && ~aVarTruthTableCondition_2 && aVarTruthTableCondition_3 && ~aVarTruthTableCondition_4)
    |     aFcnTruthTableAction_1();
    | elseif (~aVarTruthTableCondition_1 && ~aVarTruthTableCondition_2 && ~aVarTruthTableCondition_3 && aVarTruthTableCondition_4)
    |     aFcnTruthTableAction_1();
    | elseif (~aVarTruthTableCondition_1 && ~aVarTruthTableCondition_2 && ~aVarTruthTableCondition_3 && ~aVarTruthTableCondition_4 && aVarTruthTableCondition_5 && ~aVarTruthTableCondition_6 && ~aVarTruthTableCondition_8)
    |     aFcnTruthTableAction_1();
    | elseif (~aVarTruthTableCondition_1 && ~aVarTruthTableCondition_2 && ~aVarTruthTableCondition_3 && ~aVarTruthTableCondition_4 && ~aVarTruthTableCondition_5 && aVarTruthTableCondition_6 && ~aVarTruthTableCondition_7 && ~aVarTruthTableCondition_8)
    |     aFcnTruthTableAction_3();
    | elseif (~aVarTruthTableCondition_1 && ~aVarTruthTableCondition_2 && ~aVarTruthTableCondition_3 && ~aVarTruthTableCondition_4 && ~aVarTruthTableCondition_5 && ~aVarTruthTableCondition_6 && aVarTruthTableCondition_8 && ~aVarTruthTableCondition_9)
    |     aFcnTruthTableAction_1();
    | elseif (~aVarTruthTableCondition_1 && ~aVarTruthTableCondition_2 && ~aVarTruthTableCondition_3 && ~aVarTruthTableCondition_4 && ~aVarTruthTableCondition_5 && ~aVarTruthTableCondition_6 && aVarTruthTableCondition_8 && aVarTruthTableCondition_9)
    |     aFcnTruthTableAction_2();
    | else % Default
    |     aFcnTruthTableAction_1();
    | end
    | 
    | function aFcnTruthTableAction_1()
    | 
    | % Locked
    | 
    | OP_MODE = 2;
    | 
    | function aFcnTruthTableAction_2()
    | 
    | % Auto-Trim
    | 
    | OP_MODE = 3;
    | 
    | function aFcnTruthTableAction_3()
    | 
    | % Direct
    | 
    | OP_MODE = 4;
